simulink model "HANcoder_Olimexino_F3_ACC"  (R2023a)
settings: Solver=FixedStepDiscrete  StartTime=0.0  StopTime=2  FixedStep=0.01  RelTol=1e-3
PreLoadFcn:
  | librarySetup
  | eval([bdroot,'_startup']) %Calling [modelName]_startup.m
values from neighbouring files (symbols this model uses):
  b = 50    [HANcoder_Olimexino_F3_ACC_startup.m]
  m = 1000    [HANcoder_Olimexino_F3_ACC_startup.m]
undefined symbols (not defined in the file or in its folder): CON3, D3, DiscIntNeverNeededParam, F3, TIM2, USB
libraries: HANcoder_STM32_Target x10, slpidlib x2, simulink x2, simulink_extras x1, dspstat3 x1
settings Model: Creator=Jason van Kolfschoten  LastModifiedBy=joeri
settings SolverCC: AlgebraicLoopSolver=TrustRegion  PositivePriorityOrder=on
settings DataIOCC: LimitDataPoints=on  SaveFormat=Array  SignalLoggingSaveFormat=ModelDataLogs  SaveOutput=off  SaveTime=off  ReturnWorkspaceOutputs=off
settings OptimizationCC: BlockReduction=off  DefaultParameterBehavior=Inlined  DefaultUnderspecifiedDataType=single  InlineInvariantSignals=on  ExpressionDepthLimit=2147483647  StateBitsets=on  DataBitsets=on  ZeroExternalMemoryAtStartup=off  ZeroInternalMemoryAtStartup=off  InitFltsAndDblsToZero=on  NoFixptDivByZeroProtection=on  EfficientFloat2IntCast=on  LifeSpan=inf  EfficientTunableParamExpr=on
settings DebuggingCC: SaveWithDisabledLinksMsg=none  SaveWithParameterizedLinksMsg=none  CheckSSInitialOutputMsg=off  UnderspecifiedInitializationDetection=Classic  MergeDetectMultiDrivingBlocksExec=none  SignalResolutionControl=TryResolveAll  SolverPrmCheckMsg=warning  InheritedTsInSrcMsg=none  MultiTaskDSMMsg=warning  MultiTaskCondExecSysMsg=none  ParameterPrecisionLossMsg=none  FcnCallInpInsideContextMsg=warning  UnconnectedInputMsg=warning  UnconnectedOutputMsg=warning  UnconnectedLineMsg=warning  StateNameClashWarn=warning  SFUnexpectedBacktrackingDiag=warning  SFNoUnconditionalDefaultTransitionDiag=warning  SFExecutionAtInitializationDiag=none  ArithmeticOperatorsInVariantConditions=warning
settings HardwareCC: ProdBitPerPointer=32  ProdBitPerSizeT=32  ProdBitPerPtrDiffT=32  ProdLargestAtomicInteger=Long  ProdLargestAtomicFloat=Double  ProdWordSize=32  ProdHWDeviceType=ARM Compatible->ARM Cortex  TargetEndianess=LittleEndian  TargetHWDeviceType=Infineon->TriCore
settings ModelReferenceCC: EnableRefExpFcnMdlSchedulingChecks=on  PropagateSignalLabelsOutOfModel=off
settings SFSimCC: SimUseLocalCustomCode=off  MATLABDynamicMemAlloc=off  CustomCodeUndefinedFunction=UseInterfaceOnly
settings RTWCC: Description=Real-Time Workshop Embedded Coder (no auto configuration)  SystemTargetFile=ert.tlc  MakeCommand=make_rtw SHELL= HANcoder_PORTABLE=1 HANcoder_BOOTLOADER=1  TemplateMakefile=Olimexino_STM32_F3_gcc.tmf  RTWUseLocalCustomCode=off
settings CodeAppCC: ForceParamTrailComments=on  IgnoreCustomStorageClasses=off  SimulinkDataObjDesc=on  CustomSymbolStrGlobalVar=rt$N$M  CustomSymbolStrType=$N$M  CustomSymbolStrFcn=$N$M$F  CustomSymbolStrMacro=$N$M  InsertBlockDesc=on  StateflowObjectComments=on  InternalIdentifier=Classic
settings ERTTargetCC: TargetFcnLib=ansi_tfl_tmw.mat  MultiwordLength=2048  IncludeMdlTerminateFcn=off  SuppressErrorStatus=on  SupportNonFinite=off  GenerateASAP2=on  InlinedParameterPlacement=NonHierarchical  ERTCustomFileTemplate=example_file_process.tlc  ConvertIfToSwitch=off  SuppressUnreachableDefaultCases=off
settings ConfigComp: CovMetricSettings=dw  CovSaveCumulativeToWorkspaceVar=on  CovSaveSingleToWorkspaceVar=on  CovExternalEMLEnable=off  CovSFcnEnable=off  DVMaxProcessTime=600  DVAutomaticStubbing=off  DVSubSystemToStub=7.76600366011452e-316  DVParameterNames=7.76600366011452e-316  DVParameterConstraints=7.76600366011452e-316  DVParameterUseInAnalysis=7.76600366011452e-316  DVModelCoverageObjectives=MCDC  DVMaxTestCaseSteps=500  DVTestSuiteOptimization=CombinedObjectives  DVDetectActiveLogic=on  DVSaveHarnessModel=on  DVHarnessSource=Signal Editor

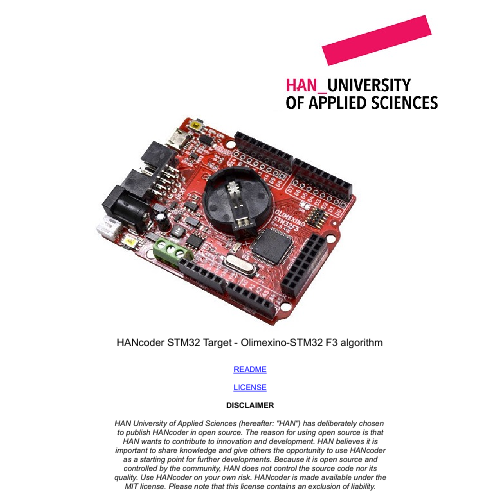
[thumbnail: Simulink's stored preview of the top-level diagram]
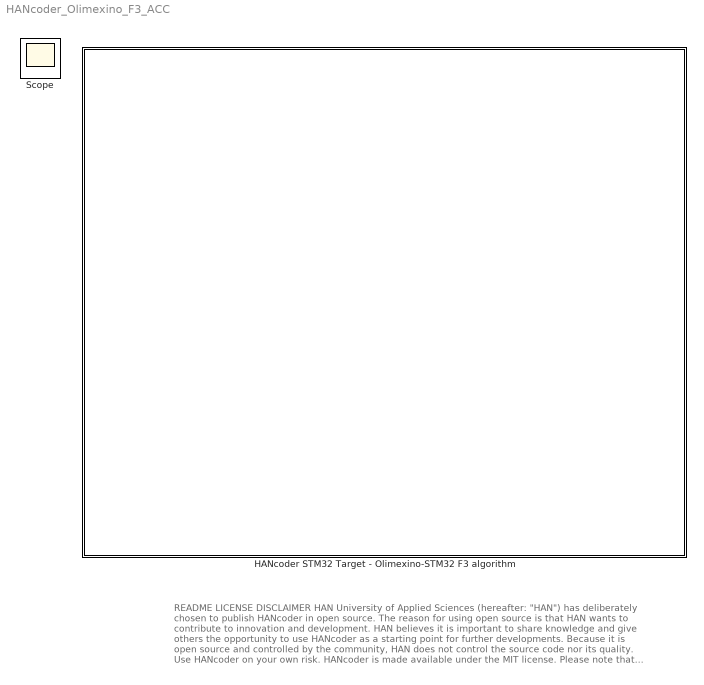
== system HANcoder_Olimexino_F3_ACC ==
  note: README
      |
      | LICENSE
      |
      | DISCLAIMER
      |
      | HAN University of Applied Sciences (hereafter: "HAN") has deliberately chosen
      | to publish HANcoder in open source. The reason for using open source is that
      | HAN wants to contribute to innovation and development. HAN believes it is
      | important to share knowledge and give others the opportunity to use HANcoder
      | as a starting point for further developments. Because it is open source and
      | controlled by the community, HAN does not control the source code nor its
      | quality. Use HANcoder on your own risk. HANcoder is made available under the
      | MIT license. Please note that this license contains an exclusion of liability.
  HANcoder STM32 Target - Olimexino-STM32 F3 algorithm : Subsystem  mask(TopLevelSubsystem){}
      mask Display: image(imread('Olimexino_STM32_F3_HAN.jpg'))
  Scope : Scope

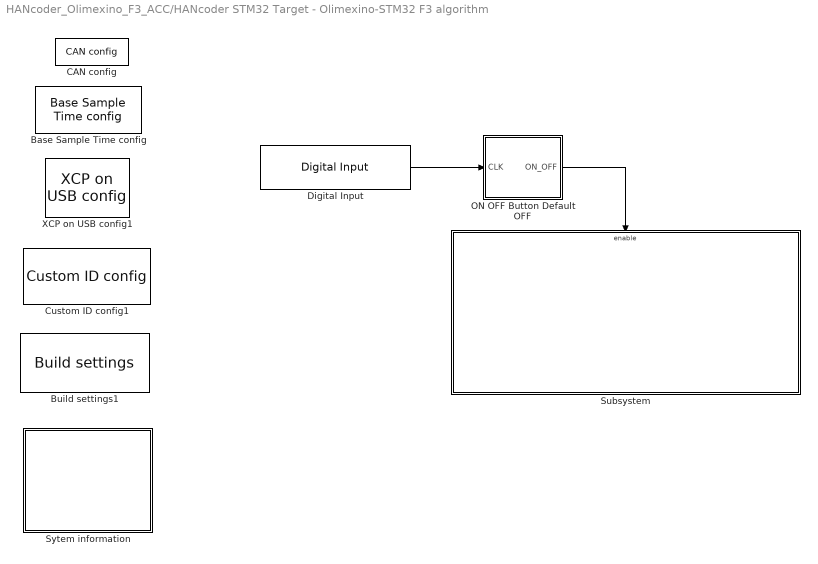
== system HANcoder_Olimexino_F3_ACC/HANcoder STM32 Target - Olimexino-STM32 F3 algorithm ==
  Base Sample Time config : HANcoder_STM32_Target/Olimexino STM32 F3/System Config/Base Sample Time config  Tag=HANcoder_TARGET_STM32_F3_Olimexino  Description=HANcoder Target STM32-Olimexino blockset version 1.2  baseSampleTime=10  extraStack=25
      settings: SourceProductName=HANcoder STM32 Target v1.2
  Build settings1 : HANcoder_STM32_Target/Olimexino STM32 F3/System Config/Build settings  Tag=HANcoder_TARGET_STM32_F3_Olimexino  AutoASAP2add=on  AutoFlash=USB-F3
      settings: SourceProductName=HANcoder STM32 Target v1.2
  CAN config : HANcoder_STM32_Target/Olimexino STM32/System Config/CAN config  Tag=HANcoder_TARGET_STM32_F3_Olimexino  canBus1=on  baudRate1=500  rxMask1=hex2dec('00000000')  rxCode1=hex2dec('00000000')  rxMode1=Receive only 11-bit message identifiers  txBufSize1=32  evBufSize1=8
      settings: SourceProductName=HANcoder STM32 Target v1.2
  Custom ID config1 : HANcoder_STM32_Target/Olimexino STM32 F3/System Config/Custom ID config  Tag=HANcoder_TARGET_STM32_F3_Olimexino  softID=softwareID  softNUM=1
      settings: SourceProductName=HANcoder STM32 Target v1.2
  Digital Input : HANcoder_STM32_Target/Olimexino STM32 F3/Digital Inputs/Digital Input  Tag=HANcoder_TARGET_STM32_F3_Olimexino  pinID=Pushbutton - BUT/BOOT0 - 5V Tolerant  config=Pulldown  tsamp=-1
      settings: SourceProductName=HANcoder STM32 Target v1.2
  ON OFF Button Default OFF : Subsystem
  Subsystem : Subsystem
  Sytem information : Subsystem
  XCP on USB config1 : HANcoder_STM32_Target/Olimexino STM32 F3/System Config/XCP on USB config  Tag=HANcoder_TARGET_STM32_F3_Olimexino
      settings: SourceProductName=HANcoder STM32 Target v1.2
  wires:
  Digital Input/1 -> ON OFF Button Default OFF/1(CLK)
  ON OFF Button Default OFF/1(ON_OFF) -> Subsystem/Enable

== system HANcoder_Olimexino_F3_ACC/HANcoder STM32 Target - Olimexino-STM32 F3 algorithm/ON OFF Button Default OFF ==
  CLK : Inport
  Constant : Constant  OutDataTypeStr=boolean
  J-K Flip-Flop : simulink_extras/Flip Flops/J-K Flip-Flop  initial_condition=0
  Signal Conversion : SignalConversion  OverrideOpt=off
  Terminator : Terminator
  ON_OFF : Outport
  wires:
  Constant/1 -> J-K Flip-Flop/3, J-K Flip-Flop/1
  J-K Flip-Flop/2 -> Terminator/1
  J-K Flip-Flop/1 -> Signal Conversion/1
  Signal Conversion/1 -> ON_OFF/1  "ON_OFF"
  CLK/1 -> J-K Flip-Flop/2

== system HANcoder_Olimexino_F3_ACC/HANcoder STM32 Target - Olimexino-STM32 F3 algorithm/Subsystem ==
  Enable : EnablePort
  Algorithm : Subsystem
  Inputs : Subsystem
  Outputs : Subsystem
  wires:
  Inputs/1(MORE vehicle speed) -> Algorithm/1(MORE Vehicle Speed)
  Inputs/4(Distance Setpoint) -> Algorithm/4(Distance setpoint CAN)
  Algorithm/1(Control effort) -> Outputs/1(Control Effort)
  Inputs/3(Speed Setpoint) -> Algorithm/3(Speed setpoint CAN)
  Inputs/2(Camera Gap) -> Algorithm/2(Distance gap)
  Inputs/5(Gap Valid) -> Algorithm/5(Gap Valid)

== system HANcoder_Olimexino_F3_ACC/HANcoder STM32 Target - Olimexino-STM32 F3 algorithm/Sytem information ==
  Get CPU load1 : HANcoder_STM32_Target/Olimexino STM32 F3/System Management/Get CPU load  Tag=HANcoder_TARGET_STM32_F3_Olimexino  mode=Current CPU load  tsamp=-1
      settings: SourceProductName=HANcoder STM32 Target v1.2
  Get free Heap1 : HANcoder_STM32_Target/Olimexino STM32 F3/System Management/Get free Heap  Tag=HANcoder_TARGET_STM32_F3_Olimexino  tsamp=-1
      settings: SourceProductName=HANcoder STM32 Target v1.2
  Get free Stack1 : HANcoder_STM32_Target/Olimexino STM32 F3/System Management/Get free Stack  Tag=HANcoder_TARGET_STM32_F3_Olimexino  taskIdx=Application Control Task  tsamp=-1
      settings: SourceProductName=HANcoder STM32 Target v1.2
  Terminator : Terminator
  Terminator1 : Terminator
  Terminator2 : Terminator
  wires:
  Get CPU load1/1 -> Terminator/1  "SI_CPUload"
  Get free Stack1/1 -> Terminator1/1  "SI_FreeStack"
  Get free Heap1/1 -> Terminator2/1  "SI_FreeHeap"

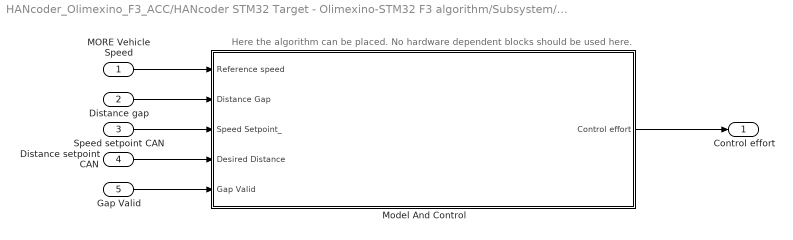
== system HANcoder_Olimexino_F3_ACC/HANcoder STM32 Target - Olimexino-STM32 F3 algorithm/Subsystem/Algorithm ==
  note: Here the algorithm can be placed. No hardware dependent blocks should be used here.
  MORE Vehicle Speed : Inport
  Distance gap : Inport  Port=2
  Speed setpoint CAN : Inport  Port=3
  Distance setpoint CAN : Inport  Port=4
  Gap Valid : Inport  Port=5
  Model And Control : Subsystem
  Control effort : Outport
  wires:
  MORE Vehicle Speed/1 -> Model And Control/1(Reference speed)
  Distance gap/1 -> Model And Control/2(Distance Gap)
  Model And Control/1(Control effort) -> Control effort/1
  Distance setpoint CAN/1 -> Model And Control/4(Desired Distance)
  Speed setpoint CAN/1 -> Model And Control/3(Speed Setpoint_)
  Gap Valid/1 -> Model And Control/5(Gap Valid)

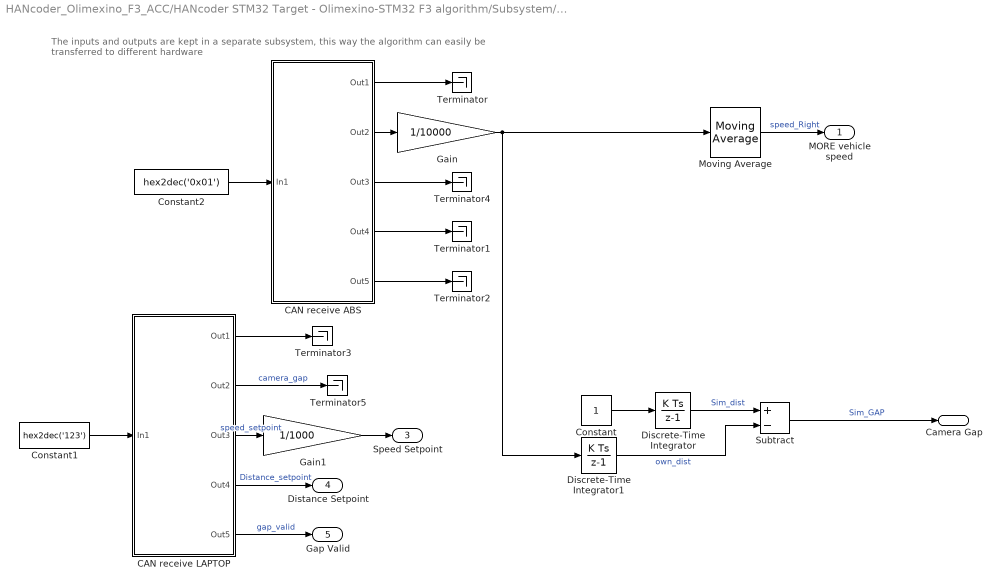
== system HANcoder_Olimexino_F3_ACC/HANcoder STM32 Target - Olimexino-STM32 F3 algorithm/Subsystem/Inputs ==
  note: The inputs and outputs are kept in a separate subsystem, this way the algorithm can easily be transferred to different hardware
  CAN receive ABS : Subsystem  Tag=HANcoder_TARGET_STM32_F3_Olimexino  AncestorBlock=HANcoder_STM32_Target/STM32-P405/CAN/CAN/CAN receive  mask(CAN receive){canBus=CAN 1, outputNumber=4, dataType=uint16, byteOrder=off, tsamp=-1}
      mask prompts: canBus "CAN channel"; outputNumber "Output ports"; dataType "Output datatype"; byteOrder "Byte order: Checked = MSB first, unchecked = LSB first."; tsamp "Sample time"
      mask help:
      | Function
      | ==========
      | Receive the newest message from the specified CAN channel.
      |
      | Parameters
      | ==========
      | CAN channel:             The CAN channel to send the message on.
      | Output ports:             The amount of output ports
      | Output datatype:       The datatype of the output ports
      | Byte order:                 Select MSB or LSB first
      | Sample time:              -1 or divisible by base sample time [seconds]
      |
      | Input
      | ==========
      | Port 1:                       CAN ID(uint32) in hexadecimal ie: hex2dec('0a')
      |
      | Output
      | ==========
      | Port 1:                       Checks for new message(int8)
      | Port 2..9                     Message data
      mask init:
      | sfcn_can_receive_mcb(canBus, outputNumber, dataType, byteOrder)
      settings: LibrarySourceBlock=HANcoder_STM32_Target/STM32-P405/CAN/CAN/CAN receive  MoveFcn=drawLogos
      mask Help: web('sfcn_can_receive.html');
      mask TypeOptions canBus: CAN 1 | CAN 2
      mask TypeOptions dataType: int8 | uint8 | int16 | uint16 | int32 | uint32 | boolean
      mask Display:
      | fprintf('Receive on\nCAN %x', canBus);
      | port_label('output', 1, 'new');
      | port_label('input', 1, 'ID');patch([79 98 97 78],[2 6 10 6],[0.89804 0 0.33725]);
  CAN receive LAPTOP : Subsystem  Tag=HANcoder_TARGET_STM32_F3_Olimexino  AncestorBlock=HANcoder_STM32_Target/STM32-P405/CAN/CAN/CAN receive  mask(CAN receive){canBus=CAN 1, outputNumber=4, dataType=int16, byteOrder=off, tsamp=-1}
      mask prompts: canBus "CAN channel"; outputNumber "Output ports"; dataType "Output datatype"; byteOrder "Byte order: Checked = MSB first, unchecked = LSB first."; tsamp "Sample time"
      mask help:
      | Function
      | ==========
      | Receive the newest message from the specified CAN channel.
      |
      | Parameters
      | ==========
      | CAN channel:             The CAN channel to send the message on.
      | Output ports:             The amount of output ports
      | Output datatype:       The datatype of the output ports
      | Byte order:                 Select MSB or LSB first
      | Sample time:              -1 or divisible by base sample time [seconds]
      |
      | Input
      | ==========
      | Port 1:                       CAN ID(uint32) in hexadecimal ie: hex2dec('0a')
      |
      | Output
      | ==========
      | Port 1:                       Checks for new message(int8)
      | Port 2..9                     Message data
      mask init:
      | sfcn_can_receive_mcb(canBus, outputNumber, dataType, byteOrder)
      settings: LibrarySourceBlock=HANcoder_STM32_Target/STM32-P405/CAN/CAN/CAN receive  MoveFcn=drawLogos
      mask Help: web('sfcn_can_receive.html');
      mask TypeOptions canBus: CAN 1 | CAN 2
      mask TypeOptions dataType: int8 | uint8 | int16 | uint16 | int32 | uint32 | boolean
      mask Display:
      | fprintf('Receive on\nCAN %x', canBus);
      | port_label('output', 1, 'new');
      | port_label('input', 1, 'ID');patch([79 98 97 78],[2 6 10 6],[0.89804 0 0.33725]);
  Constant : Constant
  Constant1 : Constant  Value=hex2dec('123')  OutDataTypeStr=uint32
  Constant2 : Constant  Value=hex2dec('0x01')  OutDataTypeStr=uint32
  Discrete-Time Integrator : DiscreteIntegrator  InitialCondition=20  SampleTime=-1  ICPrevOutput=DiscIntNeverNeededParam  ICPrevScaledInput=DiscIntNeverNeededParam
  Discrete-Time Integrator1 : DiscreteIntegrator  SampleTime=-1  OutDataTypeStr=double  ICPrevOutput=DiscIntNeverNeededParam  ICPrevScaledInput=DiscIntNeverNeededParam
  Gain : Gain  Gain=1/10000  OutDataTypeStr=double
  Gain1 : Gain  Gain=1/1000  OutDataTypeStr=double
  Moving Average : dspstat3/Moving Average  Method=Sliding window  ForgettingFactorPort=off  SpecifyWindowLength=on  WindowLength=10  OverlapLength=9  AllowArbitraryInputLength=off  ForgettingFactor=0.9  SimulateUsing=Code generation
  Subtract : Sum  Inputs=+-
  Terminator{,1..5} (6 alike) : Terminator
  MORE vehicle speed : Outport
  Camera Gap : Outport  Port=2
  Speed Setpoint : Outport  Port=3  OutDataTypeStr=double
  Distance Setpoint : Outport  Port=4
  Gap Valid : Outport  Port=5
  wires:
  Constant2/1 -> CAN receive ABS/1(In1)
  CAN receive ABS/1(Out1) -> Terminator/1
  CAN receive ABS/2(Out2) -> Gain/1
  CAN receive ABS/3(Out3) -> Terminator4/1
  CAN receive ABS/4(Out4) -> Terminator1/1
  CAN receive ABS/5(Out5) -> Terminator2/1
  CAN receive LAPTOP/1(Out1) -> Terminator3/1
  CAN receive LAPTOP/5(Out5) -> Gap Valid/1  "gap_valid"
  Constant1/1 -> CAN receive LAPTOP/1(In1)
  CAN receive LAPTOP/4(Out4) -> Distance Setpoint/1  "Distance_setpoint"
  CAN receive LAPTOP/3(Out3) -> Gain1/1  "speed_setpoint"
  Gain/1 -> Discrete-Time Integrator1/1, Moving Average/1
  Discrete-Time Integrator/1 -> Subtract/1  "Sim_dist"
  Constant/1 -> Discrete-Time Integrator/1
  CAN receive LAPTOP/2(Out2) -> Terminator5/1  "camera_gap"
  Subtract/1 -> Camera Gap/1  "Sim_GAP"
  Discrete-Time Integrator1/1 -> Subtract/2  "own_dist"
  Gain1/1 -> Speed Setpoint/1
  Moving Average/1 -> MORE vehicle speed/1  "speed_Right"

== system HANcoder_Olimexino_F3_ACC/HANcoder STM32 Target - Olimexino-STM32 F3 algorithm/Subsystem/Outputs ==
  note: The inputs and outputs are kept in a separate subsystem, this way the algorithm can easily be transferred to different hardware
  Control Effort : Inport
  PWM Duty Cycle : HANcoder_STM32_Target/Olimexino STM32 F3/PWM Outputs/PWM Duty Cycle  Tag=HANcoder_TARGET_STM32_F3_Olimexino  pinID=TIM2 - CON3 - D3  tsamp=-1
      settings: SourceProductName=HANcoder STM32 Target v1.2
  PWM Init : Subsystem  Tag=HANcoder_TARGET_STM32_F3_Olimexino  AncestorBlock=HANcoder_STM32_Target/Olimexino STM32 F3/PWM Outputs/PWM Init  mask(Pulse Width Modulation Initialization){moduleID=TIM2: D2 & D3 & n/a & D0, frequency=20, alignment=Edge aligned, enableIRQoutput=off, ch1On=off, ch1Pol=Active high, ch1Inv=off, ch2On=on, ch2Pol=Active high, ch2Inv=off, ch3On=off, ch3Pol=Active high, ch3Inv=off, ch4On=off, ch4Pol=Active high, ch4Inv=off}
      mask prompts: moduleID "PWM module"; frequency "Signal frequency [Hz]"; alignment "Signal alignment"; enableIRQoutput "Enable IRQ output"; ch1On "Generate PWM signal on channel 1"; ch1Pol "Select signal polarity"; ch1Inv "Enable inverted signal on additional output pin"; ch2On "Generate PWM signal on channel 2"; ch2Pol "Select signal polarity"; ch2Inv "Enable inverted signal on additional output pin"; ch3On "Generate PWM signal on channel 3"; ch3Pol "Select signal polarity"; ch3Inv "Enable inverted signal on additional output pin"; ch4On "Generate PWM signal on channel 4"; ch4Pol "Select signal polarity"; ch4Inv "Enable inverted signal on additional output pin"
      mask help:
      | Function
      | ========
      | A 'PWM Init' block configures one of the STM32 timer modules for PWM
      | functionality, allowing a PWM signal to be generated on up to 4 timer
      | channels and their associated output pins.
      |
      | Parameters
      | ==========
      | General - PWM module:
      |   Select the PWM module to use. The name in the combo box contains
      |   information about which pins on the target belong to this timer module.
      |   Also the first pin corresponds with the first channel and so on:
      |   TIMx: Ch1 & Ch2 & Ch3...
      |
      | General - Signal frequency:
      |   Determines the signal frequency in Hz. If you click 'Apply' after entering
      |   the desired frequency it will automatically be adjusted to the closest
      |   supported value.
      |
      | General - Signal Aligment:
      |   Determines the aligment of the signal. It can either be edge aligned or
      |   center aligned.
      |
      | General - Enable IRQ output
      |   Controls whether or not the IRQ output is available.
      |
      | Channel x - Generate PWM signal on channel x:
      |   Enable to configure the channel for PWM functionality so that the PWM signal
      |   is outputted on the channel's associated microcontroller pin.
      |
      | Channel x - Signal polarity:
      |   Selects the polarity of the signal.
      |
      | Channel x - Enable inverted signal on additional output pin:
      |   When enabled, a second PWM signal will be generated on an additional
      |   microcontroller pin where the signal is an exact inversion of the first signal.
      mask init:
      | moduleIDInfoStr = sfcn_pwmout_init_mcb(1, moduleID, frequency, alignment, enableIRQoutput, ch1On, ch2On, ch3On, ch4On, ch1Pol, ch2Pol, ch3Pol, ch4Pol, ch1Inv, ch2Inv, ch3Inv, ch4Inv);
      settings: LibrarySourceBlock=HANcoder_STM32_Target/Olimexino STM32 F3/PWM Outputs/PWM Init  CopyFcn=sfcn_pwmout_init_chk();  MoveFcn=drawLogos
      mask Help: web('sfcn_pwmout_init.html');
      mask TypeOptions moduleID: TIM1: D6 & D7 & D8 & n/a + N-channels D32 & D33 & D34  | TIM2: D2 & D3 & n/a & D0 | TIM3: D35 & D36 & D37 & n/a | TIM4: D5 & D9 & D14 & D24
      mask Callback moduleID: sfcn_pwmout_init_chk();
      mask TypeOptions alignment: Edge aligned | Center aligned
      mask TypeOptions ch1Pol: Active high | Active low
      mask TypeOptions ch2Pol: Active high | Active low
      mask TypeOptions ch3Pol: Active high | Active low
      mask TypeOptions ch4Pol: Active high | Active low
      mask Display: fprintf('PWM Init\n%s', moduleIDInfoStr);patch([214 233 232 213],[2 6 10 6],[0.89804 0 0.33725]);
  wires:
  Control Effort/1 -> PWM Duty Cycle/1

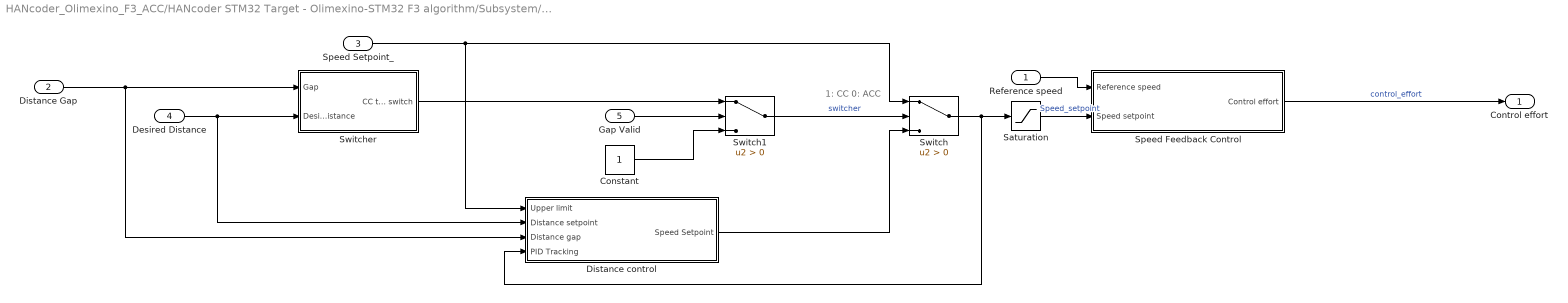
== system HANcoder_Olimexino_F3_ACC/HANcoder STM32 Target - Olimexino-STM32 F3 algorithm/Subsystem/Algorithm/Model And Control ==
  note: 1: CC
      | 0: ACC
  Reference speed : Inport
  Distance Gap : Inport  Port=2
  Speed Setpoint_ : Inport  Port=3  OutDataTypeStr=double
  Desired Distance : Inport  Port=4
  Gap Valid : Inport  Port=5
  Constant : Constant
  Distance control : Subsystem
  Saturation : Saturate  UpperLimit=3  LowerLimit=0
  Speed Feedback Control : Subsystem
  Switch : Switch  Criteria=u2 > Threshold  SaturateOnIntegerOverflow=off  InputSameDT=off
  Switch1 : Switch  Criteria=u2 > Threshold  SaturateOnIntegerOverflow=off  InputSameDT=off
  Switcher : Subsystem
  Control effort : Outport
  wires:
  Speed Setpoint_/1 -> Switch/1, Distance control/1(Upper limit)
  Speed Feedback Control/1(Control effort) -> Control effort/1  "control_effort"
  Distance control/1(Speed Setpoint) -> Switch/3
  Distance Gap/1 -> Distance control/3(Distance gap), Switcher/1(Gap)
  Switch/1 -> Distance control/4(PID Tracking), Saturation/1
  Desired Distance/1 -> Distance control/2(Distance setpoint), Switcher/2(Desired Distance)
  Reference speed/1 -> Speed Feedback Control/1(Reference speed)
  Gap Valid/1 -> Switch1/2
  Saturation/1 -> Speed Feedback Control/2(Speed setpoint)  "Speed_setpoint"
  Switcher/1(CC to ACC switch) -> Switch1/1
  Switch1/1 -> Switch/2  "switcher"
  Constant/1 -> Switch1/3

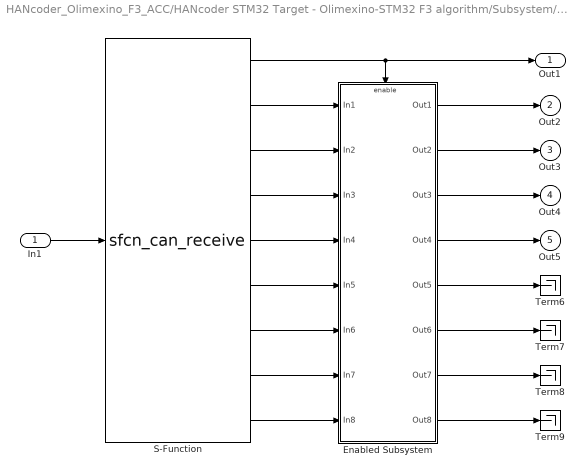
== system HANcoder_Olimexino_F3_ACC/HANcoder STM32 Target - Olimexino-STM32 F3 algorithm/Subsystem/Inputs/CAN receive ABS ==
  In1 : Inport
  Enabled Subsystem : Subsystem  TreatAsAtomicUnit=on
  S-Function : M-S-Function  FunctionName=sfcn_can_receive  Parameters=tsamp, canBus, outputNumber, dataType, byteOrder
  Term{6..9} (4 alike) : Terminator
  Out1 : Outport  VectorParamsAs1DForOutWhenUnconnected=off
  Out2 : Outport  Port=2  VectorParamsAs1DForOutWhenUnconnected=off
  Out3 : Outport  Port=3
  Out4 : Outport  Port=4
  Out5 : Outport  Port=5
  wires:
  S-Function/9 -> Enabled Subsystem/8(In8)
  S-Function/4 -> Enabled Subsystem/3(In3)
  S-Function/5 -> Enabled Subsystem/4(In4)
  S-Function/8 -> Enabled Subsystem/7(In7)
  S-Function/7 -> Enabled Subsystem/6(In6)
  S-Function/6 -> Enabled Subsystem/5(In5)
  Enabled Subsystem/8(Out8) -> Term9/1
  Enabled Subsystem/7(Out7) -> Term8/1
  Enabled Subsystem/6(Out6) -> Term7/1
  Enabled Subsystem/5(Out5) -> Term6/1
  Enabled Subsystem/4(Out4) -> Out5/1
  Enabled Subsystem/3(Out3) -> Out4/1
  Enabled Subsystem/2(Out2) -> Out3/1
  Enabled Subsystem/1(Out1) -> Out2/1
  S-Function/3 -> Enabled Subsystem/2(In2)
  S-Function/2 -> Enabled Subsystem/1(In1)
  S-Function/1 -> Enabled Subsystem/Enable, Out1/1
  In1/1 -> S-Function/1

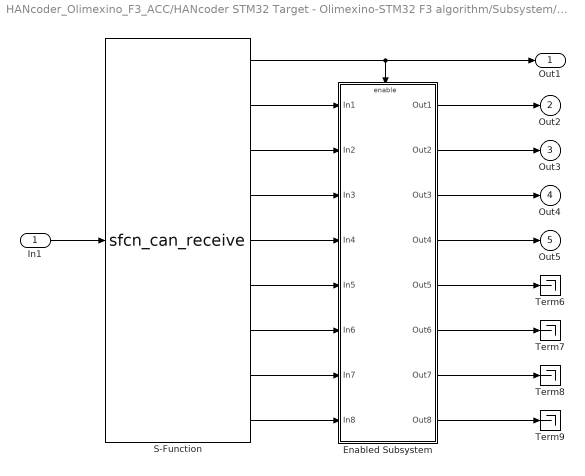
== system HANcoder_Olimexino_F3_ACC/HANcoder STM32 Target - Olimexino-STM32 F3 algorithm/Subsystem/Inputs/CAN receive LAPTOP ==
  In1 : Inport
  Enabled Subsystem : Subsystem  TreatAsAtomicUnit=on
  S-Function : M-S-Function  FunctionName=sfcn_can_receive  Parameters=tsamp, canBus, outputNumber, dataType, byteOrder
  Term{6..9} (4 alike) : Terminator
  Out1 : Outport  VectorParamsAs1DForOutWhenUnconnected=off
  Out2 : Outport  Port=2  VectorParamsAs1DForOutWhenUnconnected=off
  Out3 : Outport  Port=3
  Out4 : Outport  Port=4
  Out5 : Outport  Port=5
  wires:
  S-Function/9 -> Enabled Subsystem/8(In8)
  S-Function/4 -> Enabled Subsystem/3(In3)
  S-Function/5 -> Enabled Subsystem/4(In4)
  S-Function/8 -> Enabled Subsystem/7(In7)
  S-Function/7 -> Enabled Subsystem/6(In6)
  S-Function/6 -> Enabled Subsystem/5(In5)
  Enabled Subsystem/8(Out8) -> Term9/1
  Enabled Subsystem/7(Out7) -> Term8/1
  Enabled Subsystem/6(Out6) -> Term7/1
  Enabled Subsystem/5(Out5) -> Term6/1
  Enabled Subsystem/4(Out4) -> Out5/1
  Enabled Subsystem/3(Out3) -> Out4/1
  Enabled Subsystem/2(Out2) -> Out3/1
  Enabled Subsystem/1(Out1) -> Out2/1
  S-Function/3 -> Enabled Subsystem/2(In2)
  S-Function/2 -> Enabled Subsystem/1(In1)
  S-Function/1 -> Enabled Subsystem/Enable, Out1/1
  In1/1 -> S-Function/1

== system HANcoder_Olimexino_F3_ACC/HANcoder STM32 Target - Olimexino-STM32 F3 algorithm/Subsystem/Outputs/PWM Init ==
  S-Function : S-Function  FunctionName=sfcn_pwmout_init  SFunctionDeploymentMode=off  EnableBusSupport=off
  Term1 : Terminator
  wires:
  S-Function/1 -> Term1/1

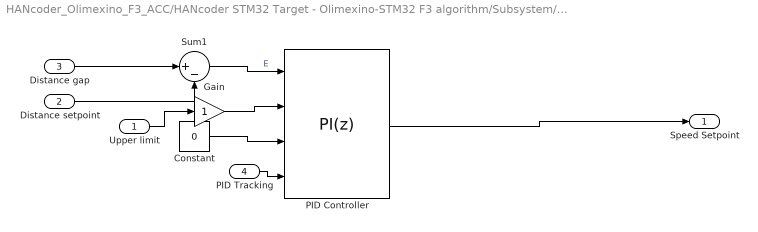
== system HANcoder_Olimexino_F3_ACC/HANcoder STM32 Target - Olimexino-STM32 F3 algorithm/Subsystem/Algorithm/Model And Control/Distance control ==
  Upper limit : Inport
  Distance setpoint : Inport  Port=2
  Distance gap : Inport  Port=3
  PID Tracking : Inport  Port=4
  Constant : Constant  Value=0
  Gain : Gain  OutDataTypeStr=double
  PID Controller : slpidlib/PID Controller  Controller=PI  Form=Parallel  TimeDomain=Discrete-time  UseExternalTs=off  SampleTime=-1  IntegratorMethod=Forward Euler  FilterMethod=Forward Euler  ControllerParametersSource=internal  P=1  I=0.1  UseKiTs=on  D=2  N=100  UseFilter=on  TunerSelectOption=Frequency Response Based  InitialConditionSource=internal  InitialConditionForIntegrator=0  InitialConditionForFilter=0  DifferentiatorICPrevScaledInput=0  ExternalReset=none  TrackingMode=on  Kt=1  LimitOutput=on  SatLimitsSource=external  UpperSaturationLimit=5000  LowerSaturationLimit=-5000  LinearizeAsGain=on  AntiWindupMode=clamping  Kb=1  LimitIntegrator=off  UpperIntegratorSaturationLimit=inf  LowerIntegratorSaturationLimit=-inf  POutMin=[]  POutMax=[]  IOutMin=[]  IOutMax=[]  DOutMin=[]  DOutMax=[]  NOutMin=[]  NOutMax=[]  SumOutMin=[]  SumOutMax=[]  SaturationOutMin=[]  SaturationOutMax=[]  PParamMin=[]  PParamMax=[]  IParamMin=[]  IParamMax=[]  DParamMin=[]  DParamMax=[]  NParamMin=[]  NParamMax=[]  KbParamMin=[]  KbParamMax=[]  KtParamMin=[]  KtParamMax=[]  KbOutMin=[]  KbOutMax=[]  KtOutMin=[]  KtOutMax=[]  IntegratorOutMin=[]  IntegratorOutMax=[]  FilterOutMin=[]  FilterOutMax=[]  SumI1OutMin=[]  SumI1OutMax=[]  SumI2OutMin=[]  SumI2OutMax=[]  SumI3OutMin=[]  SumI3OutMax=[]  SumI4OutMin=[]  SumI4OutMax=[]  SumDOutMin=[]  SumDOutMax=[]  DifferentiatorOutMin=[]  DifferentiatorOutMax=[]  FilterDiffOutCoefMin=[]  FilterDiffOutCoefMax=[]  ReciprocalOutMin=[]  ReciprocalOutMax=[]  SumDenOutMin=[]  SumDenOutMax=[]  SumNumOutMin=[]  SumNumOutMax=[]  DivideOutMin=[]  DivideOutMax=[]  UdiffTsProdOutMin=[]  UdiffTsProdOutMax=[]  NTsProdOutMin=[]  NTsProdOutMax=[]  UintegralTsProdOutMin=[]  UintegralTsProdOutMax=[]  UngainTsProdOutMin=[]  UngainTsProdOutMax=[]  ClampingZeroOutDataTypeStr=Inherit: Inherit via back propagation  ClampingZeroOutMin=[]  ClampingZeroOutMax=[]  FilterDenConstantOutDataTypeStr=Inherit: Inherit via back propagation  FilterDenConstantOutMin=[]  FilterDenConstantOutMax=[]  PCopyOutDataTypeStr=Inherit: Inherit via back propagation  PCopyOutMin=[]  PCopyOutMax=[]  NCopyOutDataTypeStr=Inherit: Inherit via back propagation  NCopyOutMin=[]  NCopyOutMax=[]  IntegratorContinuousStateAttributes=''  IntegratorStateMustResolveToSignalObject=off  IntegratorRTWStateStorageClass=Auto  FilterContinuousStateAttributes=''  FilterStateMustResolveToSignalObject=off  FilterRTWStateStorageClass=Auto  ParallelPVariant=InternalParameters  IdealPVariant=Disabled  IVariant=InternalParameters  DVariant=Disabled  IntegratorVariant=Discrete  SatVariant=External  AWVariant=DiscClampingParallel  PCopyVariant=Disabled  TRVariant=Enabled  FdbkBlocksVariant=Forward  IdealPFdbkVariant=Disabled  SatFdbkVariant=Disabled  DerivativeFilterVariant=Disabled  NVariant=Disabled  NCopyVariant=Disabled_SignalSpec  FilterICVariant=Disabled  IntegratorICVariant=InternalICs  ExternalResetVariant=Disabled  TRSumVariant=TrackingMode  SumFdbkVariant=Disabled  SumVariant=Sum_PI  TsampFilterVariant=InternalTs  TsampNgainVariant=Passthrough  TsampIntegralVariant=Disabled_SignalSpec  ExternalSaturationOutDataTypeStr=Inherit: Same as second input
  Sum1 : Sum  Inputs=|+-  AccumDataTypeStr=double
  Speed Setpoint : Outport
  wires:
  Sum1/1 -> PID Controller/1  "E"
  PID Controller/1 -> Speed Setpoint/1
  Upper limit/1 -> Gain/1
  Constant/1 -> PID Controller/3
  PID Tracking/1 -> PID Controller/4
  Distance gap/1 -> Sum1/1
  Distance setpoint/1 -> Sum1/2
  Gain/1 -> PID Controller/2

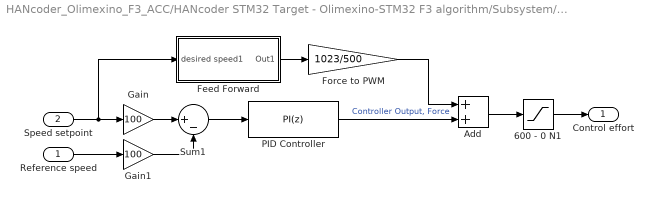
== system HANcoder_Olimexino_F3_ACC/HANcoder STM32 Target - Olimexino-STM32 F3 algorithm/Subsystem/Algorithm/Model And Control/Speed Feedback Control ==
  Reference speed : Inport
  Speed setpoint : Inport  Port=2
  600 - 0 N1 : Saturate  UpperLimit=600  LowerLimit=0  OutDataTypeStr=uint16
  Add : Sum
  Feed Forward : Subsystem
  Force to PWM : Gain  Gain=1023/500  OutDataTypeStr=int16
  Gain : Gain  Gain=100
  Gain1 : Gain  Gain=100
  PID Controller : slpidlib/PID Controller  Controller=PI  Form=Parallel  TimeDomain=Discrete-time  UseExternalTs=off  SampleTime=-1  IntegratorMethod=Forward Euler  FilterMethod=Forward Euler  ControllerParametersSource=internal  P=1  I=0.7  UseKiTs=off  D=0  N=100  UseFilter=off  TunerSelectOption=Frequency Response Based  InitialConditionSource=internal  InitialConditionForIntegrator=0  InitialConditionForFilter=0  DifferentiatorICPrevScaledInput=0  ExternalReset=none  TrackingMode=off  Kt=0  LimitOutput=on  SatLimitsSource=internal  UpperSaturationLimit=600  LowerSaturationLimit=0  LinearizeAsGain=on  AntiWindupMode=clamping  Kb=1  LimitIntegrator=off  UpperIntegratorSaturationLimit=inf  LowerIntegratorSaturationLimit=-inf  POutMin=[]  POutMax=[]  IOutMin=[]  IOutMax=[]  DOutMin=[]  DOutMax=[]  NOutMin=[]  NOutMax=[]  SumOutMin=[]  SumOutMax=[]  SaturationOutMin=[]  SaturationOutMax=[]  PParamMin=[]  PParamMax=[]  IParamMin=[]  IParamMax=[]  DParamMin=[]  DParamMax=[]  NParamMin=[]  NParamMax=[]  KbParamMin=[]  KbParamMax=[]  KtParamMin=[]  KtParamMax=[]  KbOutMin=[]  KbOutMax=[]  KtOutMin=[]  KtOutMax=[]  IntegratorOutMin=[]  IntegratorOutMax=[]  FilterOutMin=[]  FilterOutMax=[]  SumI1OutMin=[]  SumI1OutMax=[]  SumI2OutMin=[]  SumI2OutMax=[]  SumI3OutMin=[]  SumI3OutMax=[]  SumI4OutMin=[]  SumI4OutMax=[]  SumDOutMin=[]  SumDOutMax=[]  DifferentiatorOutMin=[]  DifferentiatorOutMax=[]  FilterDiffOutCoefMin=[]  FilterDiffOutCoefMax=[]  ReciprocalOutMin=[]  ReciprocalOutMax=[]  SumDenOutMin=[]  SumDenOutMax=[]  SumNumOutMin=[]  SumNumOutMax=[]  DivideOutMin=[]  DivideOutMax=[]  UdiffTsProdOutMin=[]  UdiffTsProdOutMax=[]  NTsProdOutMin=[]  NTsProdOutMax=[]  UintegralTsProdOutMin=[]  UintegralTsProdOutMax=[]  UngainTsProdOutMin=[]  UngainTsProdOutMax=[]  ClampingZeroOutDataTypeStr=Inherit: Inherit via back propagation  ClampingZeroOutMin=[]  ClampingZeroOutMax=[]  FilterDenConstantOutDataTypeStr=Inherit: Inherit via back propagation  FilterDenConstantOutMin=[]  FilterDenConstantOutMax=[]  PCopyOutDataTypeStr=Inherit: Inherit via back propagation  PCopyOutMin=[]  PCopyOutMax=[]  NCopyOutDataTypeStr=Inherit: Inherit via back propagation  NCopyOutMin=[]  NCopyOutMax=[]  IntegratorContinuousStateAttributes=''  IntegratorStateMustResolveToSignalObject=off  IntegratorRTWStateStorageClass=Auto  FilterContinuousStateAttributes=''  FilterStateMustResolveToSignalObject=off  FilterRTWStateStorageClass=Auto  ParallelPVariant=InternalParameters  IdealPVariant=Disabled  IVariant=InternalParameters  DVariant=Disabled  IntegratorVariant=Discrete  SatVariant=Enabled  AWVariant=DiscClampingParallel  PCopyVariant=Disabled  TRVariant=Disabled  FdbkBlocksVariant=Forward  IdealPFdbkVariant=Disabled  SatFdbkVariant=Disabled  DerivativeFilterVariant=Disabled  NVariant=Disabled  NCopyVariant=Disabled_SignalSpec  FilterICVariant=Disabled  IntegratorICVariant=InternalICs  ExternalResetVariant=Disabled  TRSumVariant=Passthrough  SumFdbkVariant=Disabled  SumVariant=Sum_PI  TsampFilterVariant=InternalTs  TsampNgainVariant=Passthrough  TsampIntegralVariant=Disabled_SignalSpec  ExternalSaturationOutDataTypeStr=Inherit: Same as second input
  Sum1 : Sum  Inputs=|+-
  Control effort : Outport
  wires:
  Sum1/1 -> PID Controller/1
  Speed setpoint/1 -> Gain/1, Feed Forward/1(desired speed1)
  Add/1 -> 600 - 0 N1/1
  Feed Forward/1(Out1) -> Force to PWM/1
  PID Controller/1 -> Add/2  "Controller Output, Force"
  Reference speed/1 -> Gain1/1
  Force to PWM/1 -> Add/1
  600 - 0 N1/1 -> Control effort/1
  Gain/1 -> Sum1/1
  Gain1/1 -> Sum1/2

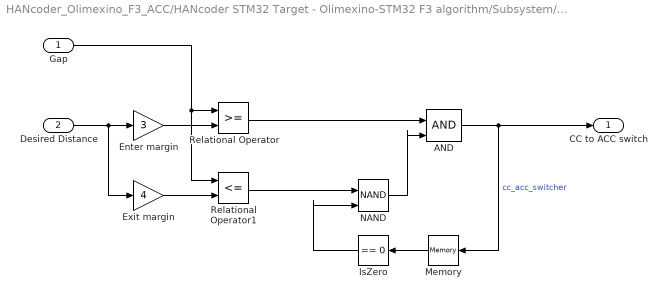
== system HANcoder_Olimexino_F3_ACC/HANcoder STM32 Target - Olimexino-STM32 F3 algorithm/Subsystem/Algorithm/Model And Control/Switcher ==
  Gap : Inport
  Desired Distance : Inport  Port=2
  AND : Logic  IconShape=distinctive  AllPortsSameDT=off  OutDataTypeStr=boolean
  Enter margin : Gain  Gain=3
  Exit margin : Gain  Gain=4
  IsZero : simulink/Logic and Bit Operations/Compare To Zero  relop===  OutDataTypeStr=boolean
  Memory : Memory
  NAND : Logic  Operator=NAND  IconShape=distinctive  AllPortsSameDT=off  OutDataTypeStr=boolean
  Relational Operator : RelationalOperator  OutDataTypeStr=boolean  RndMeth=Simplest  InputSameDT=off
  Relational Operator1 : RelationalOperator  Operator=<=  OutDataTypeStr=boolean  RndMeth=Simplest  InputSameDT=off
  CC to ACC switch : Outport
  wires:
  Enter margin/1 -> Relational Operator/2
  Desired Distance/1 -> Exit margin/1, Enter margin/1
  Exit margin/1 -> Relational Operator1/2
  Relational Operator/1 -> AND/1
  Relational Operator1/1 -> NAND/1
  Memory/1 -> IsZero/1
  NAND/1 -> AND/2
  AND/1 -> Memory/1, CC to ACC switch/1  "cc_acc_switcher"
  IsZero/1 -> NAND/2
  Gap/1 -> Relational Operator1/1, Relational Operator/1

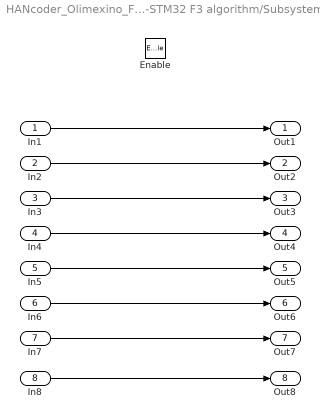
== system HANcoder_Olimexino_F3_ACC/HANcoder STM32 Target - Olimexino-STM32 F3 algorithm/Subsystem/Inputs/CAN receive ABS/Enabled Subsystem ==
  In1 : Inport
  In2 : Inport  Port=2
  In3 : Inport  Port=3
  In4 : Inport  Port=4
  In5 : Inport  Port=5
  In6 : Inport  Port=6
  In7 : Inport  Port=7
  In8 : Inport  Port=8
  Enable : EnablePort
  Out1 : Outport  VectorParamsAs1DForOutWhenUnconnected=off
  Out2 : Outport  Port=2  VectorParamsAs1DForOutWhenUnconnected=off
  Out3 : Outport  Port=3  VectorParamsAs1DForOutWhenUnconnected=off
  Out4 : Outport  Port=4  VectorParamsAs1DForOutWhenUnconnected=off
  Out5 : Outport  Port=5  VectorParamsAs1DForOutWhenUnconnected=off
  Out6 : Outport  Port=6  VectorParamsAs1DForOutWhenUnconnected=off
  Out7 : Outport  Port=7  VectorParamsAs1DForOutWhenUnconnected=off
  Out8 : Outport  Port=8  VectorParamsAs1DForOutWhenUnconnected=off
  wires:
  In8/1 -> Out8/1
  In7/1 -> Out7/1
  In6/1 -> Out6/1
  In5/1 -> Out5/1
  In4/1 -> Out4/1
  In3/1 -> Out3/1
  In2/1 -> Out2/1
  In1/1 -> Out1/1

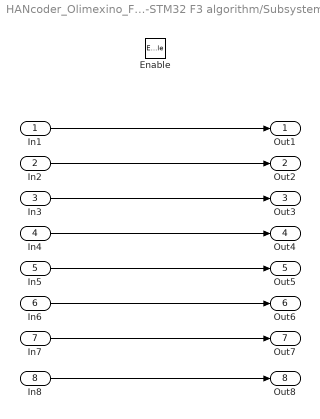
== system HANcoder_Olimexino_F3_ACC/HANcoder STM32 Target - Olimexino-STM32 F3 algorithm/Subsystem/Inputs/CAN receive LAPTOP/Enabled Subsystem ==
  In1 : Inport
  In2 : Inport  Port=2
  In3 : Inport  Port=3
  In4 : Inport  Port=4
  In5 : Inport  Port=5
  In6 : Inport  Port=6
  In7 : Inport  Port=7
  In8 : Inport  Port=8
  Enable : EnablePort
  Out1 : Outport  VectorParamsAs1DForOutWhenUnconnected=off
  Out2 : Outport  Port=2  VectorParamsAs1DForOutWhenUnconnected=off
  Out3 : Outport  Port=3  VectorParamsAs1DForOutWhenUnconnected=off
  Out4 : Outport  Port=4  VectorParamsAs1DForOutWhenUnconnected=off
  Out5 : Outport  Port=5  VectorParamsAs1DForOutWhenUnconnected=off
  Out6 : Outport  Port=6  VectorParamsAs1DForOutWhenUnconnected=off
  Out7 : Outport  Port=7  VectorParamsAs1DForOutWhenUnconnected=off
  Out8 : Outport  Port=8  VectorParamsAs1DForOutWhenUnconnected=off
  wires:
  In8/1 -> Out8/1
  In7/1 -> Out7/1
  In6/1 -> Out6/1
  In5/1 -> Out5/1
  In4/1 -> Out4/1
  In3/1 -> Out3/1
  In2/1 -> Out2/1
  In1/1 -> Out1/1

== system HANcoder_Olimexino_F3_ACC/HANcoder STM32 Target - Olimexino-STM32 F3 algorithm/Subsystem/Algorithm/Model And Control/Speed Feedback Control/Feed Forward ==
  desired speed1 : Inport
  Add : Sum
  Discrete Derivative : simulink/Discrete/Discrete Derivative  gainval=1.0  ICPrevScaledInput=0.0  OutMin=[]  OutMax=[]  OutDataType=fixdt(1, 16)  OutScaling=2^-10  DoSatur=off
  Gain : Gain  Gain=b
  Gain1 : Gain  Gain=m
  Scope : Scope
  Out1 : Outport
  wires:
  Gain/1 -> Add/2
  Discrete Derivative/1 -> Gain1/1
  desired speed1/1 -> Discrete Derivative/1, Gain/1, Scope/1
  Add/1 -> Out1/1
  Gain1/1 -> Add/1
